simulink model "counter_block_diagram"  (R2016b)
settings: Solver=VariableStepAuto  StartTime=0.0  StopTime=10.0  RelTol=1e-3
settings Model: Creator=Lupus  LastModifiedBy=Lupus

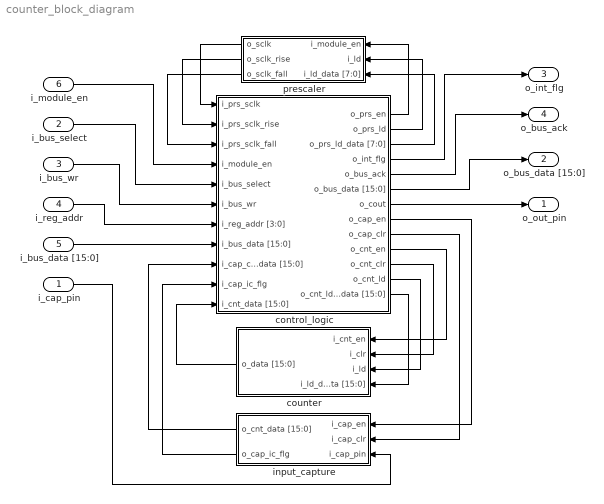
== system counter_block_diagram ==
  i_cap_pin : Inport
  i_bus_select : Inport  Port=2
  i_bus_wr : Inport  Port=3
  i_reg_addr : Inport  Port=4
  i_bus_data [15:0] : Inport  Port=5
  i_module_en : Inport  Port=6
  "control_logic " : Subsystem
  counter : Subsystem
  input_capture : Subsystem
  prescaler : Subsystem
  o_out_pin : Outport
  o_bus_data [15:0] : Outport  Port=2
  o_int_flg : Outport  Port=3
  o_bus_ack : Outport  Port=4
  wires:
  "control_logic "/1(o_prs_en) -> prescaler/1(i_module_en)
  "control_logic "/2(o_prs_ld) -> prescaler/2(i_ld)
  "control_logic "/3(o_prs_ld_data [7:0]) -> prescaler/3(i_ld_data [7:0])
  i_module_en/1 -> "control_logic "/4(i_module_en)
  i_bus_select/1 -> "control_logic "/5(i_bus_select)
  i_bus_wr/1 -> "control_logic "/6(i_bus_wr)
  i_reg_addr/1 -> "control_logic "/7(i_reg_addr [3:0])
  i_bus_data [15:0]/1 -> "control_logic "/8(i_bus_data [15:0])
  prescaler/1(o_sclk) -> "control_logic "/1(i_prs_sclk)
  prescaler/2(o_sclk_rise) -> "control_logic "/2(i_prs_sclk_rise)
  prescaler/3(o_sclk_fall) -> "control_logic "/3(i_prs_sclk_fall)
  counter/1(o_data [15:0]) -> "control_logic "/11(i_cnt_data [15:0])
  "control_logic "/13(o_cnt_ld_data [15:0]) -> counter/4(i_ld_data [15:0])
  "control_logic "/12(o_cnt_ld) -> counter/3(i_ld)
  "control_logic "/11(o_cnt_clr) -> counter/2(i_clr)
  "control_logic "/10(o_cnt_en) -> counter/1(i_cnt_en)
  input_capture/1(o_cnt_data [15:0]) -> "control_logic "/9(i_cap_cnt_data [15:0])
  input_capture/2(o_cap_ic_flg) -> "control_logic "/10(i_cap_ic_flg)
  "control_logic "/8(o_cap_en) -> input_capture/1(i_cap_en)
  "control_logic "/9(o_cap_clr) -> input_capture/2(i_cap_clr)
  i_cap_pin/1 -> input_capture/3(i_cap_pin)
  "control_logic "/4(o_int_flg) -> o_int_flg/1
  "control_logic "/5(o_bus_ack) -> o_bus_ack/1
  "control_logic "/6(o_bus_data [15:0]) -> o_bus_data [15:0]/1
  "control_logic "/7(o_cout) -> o_out_pin/1

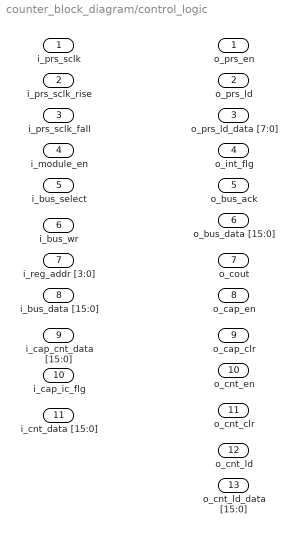
== system counter_block_diagram/control_logic  ==
  i_prs_sclk : Inport
  i_prs_sclk_rise : Inport  Port=2
  i_prs_sclk_fall : Inport  Port=3
  i_module_en : Inport  Port=4
  i_bus_select : Inport  Port=5
  i_bus_wr : Inport  Port=6
  i_reg_addr [3:0] : Inport  Port=7
  i_bus_data [15:0] : Inport  Port=8
  i_cap_cnt_data [15:0] : Inport  Port=9
  i_cap_ic_flg : Inport  Port=10
  i_cnt_data [15:0] : Inport  Port=11
  o_prs_en : Outport
  o_prs_ld : Outport  Port=2
  o_prs_ld_data [7:0] : Outport  Port=3
  o_int_flg : Outport  Port=4
  o_bus_ack : Outport  Port=5
  o_bus_data [15:0] : Outport  Port=6
  o_cout : Outport  Port=7
  o_cap_en : Outport  Port=8
  o_cap_clr : Outport  Port=9
  o_cnt_en : Outport  Port=10
  o_cnt_clr : Outport  Port=11
  o_cnt_ld : Outport  Port=12
  o_cnt_ld_data [15:0] : Outport  Port=13

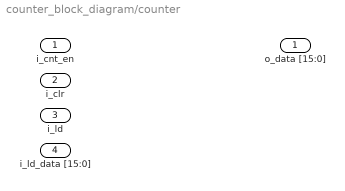
== system counter_block_diagram/counter ==
  i_cnt_en : Inport
  i_clr : Inport  Port=2
  i_ld : Inport  Port=3
  i_ld_data [15:0] : Inport  Port=4
  o_data [15:0] : Outport

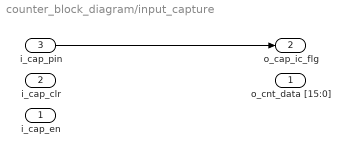
== system counter_block_diagram/input_capture ==
  i_cap_en : Inport
  i_cap_clr : Inport  Port=2
  i_cap_pin : Inport  Port=3
  o_cnt_data [15:0] : Outport
  o_cap_ic_flg : Outport  Port=2
  wires:
  i_cap_pin/1 -> o_cap_ic_flg/1

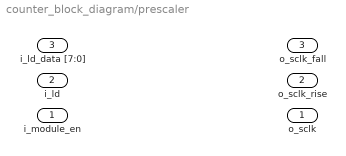
== system counter_block_diagram/prescaler ==
  i_module_en : Inport
  i_ld : Inport  Port=2
  i_ld_data [7:0] : Inport  Port=3
  o_sclk : Outport
  o_sclk_rise : Outport  Port=2
  o_sclk_fall : Outport  Port=3
